simulink model "Problem1_Mod5Counter"  (R2020b)
settings: Solver=VariableStepAuto  StartTime=0.0  StopTime=inf  RelTol=1e-3
settings Model: EnablePacing=on  PacingRate=1.800000  Creator=vigne  LastModifiedBy=prabhudevmaddipudi

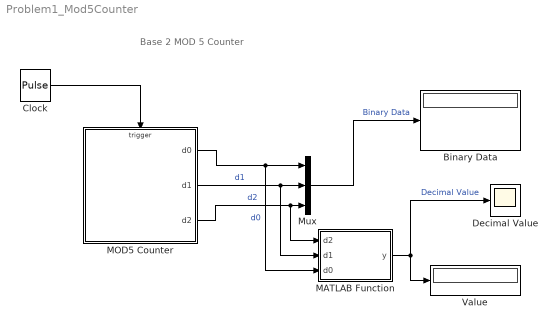
== system Problem1_Mod5Counter ==
  note: Base 2 MOD 5 Counter
  Binary Data : Display
  Clock : DiscretePulseGenerator  PulseType=Time based  Period=0.5  PulseWidth=5
  Decimal Value : Scope
  MATLAB Function : MATLAB Function  TreatAsAtomicUnit=on
  MOD5 Counter : Stateflow chart  TreatAsAtomicUnit=on
  Mux : Mux  Inputs=3
  Value : Display
  wires:
  Clock/1 -> MOD5 Counter/Trigger
  Mux/1 -> Binary Data/1  "Binary Data"
  MOD5 Counter/1(d0) -> MATLAB Function/3(d0), Mux/1  "d0"
  MOD5 Counter/2(d1) -> MATLAB Function/2(d1), Mux/2  "d1"
  MATLAB Function/1(y) -> Value/1, Decimal Value/1  "Decimal Value"
  MOD5 Counter/3(d2) -> MATLAB Function/1(d2), Mux/3  "d2"

== matlab function Problem1_Mod5Counter/MATLAB Function ==
  data: d2 input; y output; d1 input; d0 input
function y= fcn(d2,d1,d0)
if(d2==0 && d1==0 && d0==0)
    y=0;
elseif(d2==0 && d1==0 && d0==1)
    y=1;
elseif(d2==0 && d1==1 && d0==0)
    y=2;
elseif(d2==0 && d1==1 && d0==1)
    y=3;
elseif(d2==1 && d1==0 && d0==0)
    y=4;
else
    y=0;
    
end

== stateflow chart Problem1_Mod5Counter/MOD5 Counter ==
  state digit0 [parallel]
    settings: executionOrder=2
    state zero
      en:
      d0=0;
    state one
      en:
      d0=1
    (default) -> digit0.zero
    digit0.one -> digit0.zero : pulse{send(inc1);}
    digit0.zero -> digit0.one : [r==0]
  note: 000-0
      | 001-1
      | 010-2
      | 011-3
      | 100-4
      | 101-5
      | 110-6
      | 111-7
  state digit1 [parallel]
    settings: executionOrder=3
    state zero
      en:
      d1=0;
    state one
      en:
      d1=1;
    (default) -> digit1.zero
    digit1.one -> digit1.zero : inc1{send(inc2);}
    digit1.zero -> digit1.one : inc1
  state digit2 [parallel]
    settings: executionOrder=1
    state zero
      en:
      d2=0;
      du:
      r=0;
    state one
      en:
      d2=1;
      r=1;
    (default) -> digit2.zero
    digit2.one -> digit2.zero
    digit2.zero -> digit2.one : inc2
  data: d0 output; d1 output; d2 output; r local =0
  events: pulse input RISING_EDGE_EVENT; inc1 local FUNCTION_CALL_EVENT; inc2 local FUNCTION_CALL_EVENT
